simulink model "simulink_modelQ1"  (R2023a)
settings: Solver=FixedStepAuto  StartTime=0.0  StopTime=simulation_end_time  FixedStep=integration_step_time  RelTol=1e-3
values from neighbouring files (symbols this model uses):
  myu = 398603    [main.m]
  r_0_vector = [-2.1 4.2 6.5]*10^3    [main.m]
  v_0_vector = [-6.8 -1.5 -0.43]    [main.m]
undefined symbols (not defined in the file or in its folder): magnitude
settings Model: Creator=אלמוג  LastModifiedBy=אלמוג

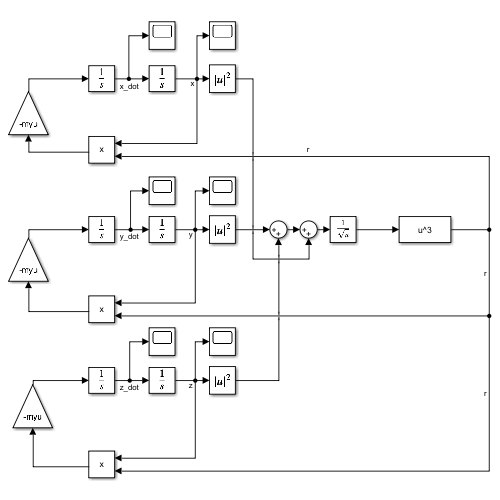
[thumbnail: Simulink's stored preview of the top-level diagram]
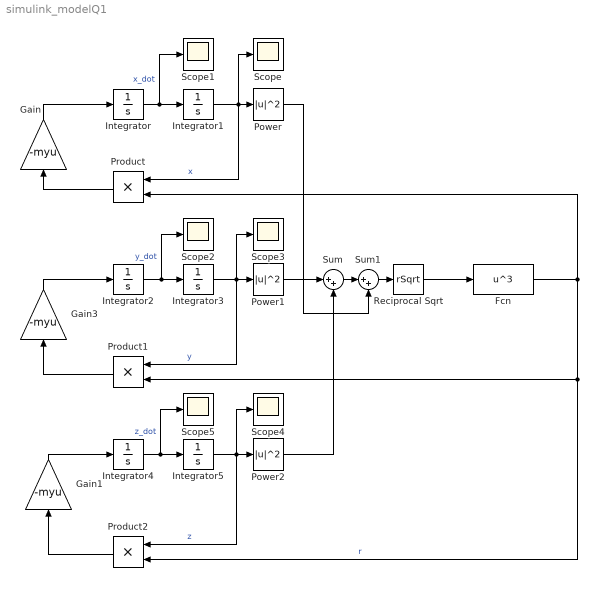
== system simulink_modelQ1 ==
  Fcn : Fcn  Expr=u^3
  Gain : Gain  Gain=-myu
  Gain1 : Gain  Gain=-myu
  Gain3 : Gain  Gain=-myu
  Integrator : Integrator  InitialCondition=v_0_vector(1)
  Integrator1 : Integrator  InitialCondition=r_0_vector(1)
  Integrator2 : Integrator  InitialCondition=v_0_vector(2)
  Integrator3 : Integrator  InitialCondition=r_0_vector(2)
  Integrator4 : Integrator  InitialCondition=v_0_vector(3)
  Integrator5 : Integrator  InitialCondition=r_0_vector(3)
  Power : Math  Operator=magnitude^2
  Power1 : Math  Operator=magnitude^2
  Power2 : Math  Operator=magnitude^2
  Product : Product
  Product1 : Product
  Product2 : Product
  Reciprocal Sqrt : Sqrt  Operator=rSqrt
  Scope{,1..5} (6 alike) : Scope
  Sum : Sum  Inputs=|++
  Sum1 : Sum  Inputs=|++
  wires:
  Gain/1 -> Integrator/1
  Integrator2/1 -> Scope2/1, Integrator3/1  "y_dot"
  Integrator3/1 -> Power1/1, Product1/1, Scope3/1  "y"
  Gain3/1 -> Integrator2/1
  Product2/1 -> Gain1/1
  Integrator5/1 -> Power2/1, Product2/1, Scope4/1  "z"
  Gain1/1 -> Integrator4/1
  Product1/1 -> Gain3/1
  Product/1 -> Gain/1
  Integrator/1 -> Scope1/1, Integrator1/1  "x_dot"
  Integrator4/1 -> Scope5/1, Integrator5/1  "z_dot"
  Integrator1/1 -> Power/1, Product/1, Scope/1  "x"
  Fcn/1 -> Product/2, Product2/2, Product1/2  "r"
  Power/1 -> Sum1/2
  Power1/1 -> Sum/1
  Power2/1 -> Sum/2
  Reciprocal Sqrt/1 -> Fcn/1
  Sum/1 -> Sum1/1
  Sum1/1 -> Reciprocal Sqrt/1
